simulink model "tiremodel_TUM"  (R2018b)
settings: configuration reference "Physics" (kept outside this file)
model workspace (MAT data in the model file):
  x0_initialstates = Simulink.Parameter
  x0_initialstates.Value = [0 0 0 0 0 0]
  x0_initialstates.DataType = 'auto'
  x0_initialstates.Dimensions = [1 6]
settings Model: DataDictionary=vehicleparameters_vehdynsim.sldd  ParameterArgumentNames=x0_initialstates  OrderedModelArguments=off  Creator=wischnewski  LastModifiedBy=ga25xiw

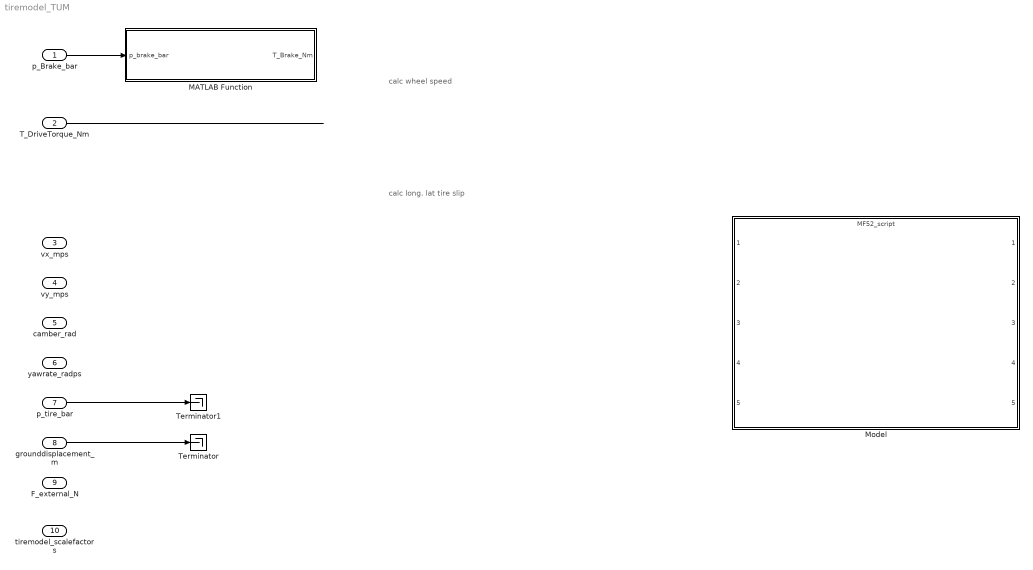
== system tiremodel_TUM ==
  note: calc wheel speed
  note: calc long. lat tire slip
  p_Brake_bar : Inport
  T_DriveTorque_Nm : Inport  Port=2
  vx_mps : Inport  Port=3
  vy_mps : Inport  Port=4
  camber_rad : Inport  Port=5
  yawrate_radps : Inport  Port=6
  p_tire_bar : Inport  Port=7
  grounddisplacement_m : Inport  Port=8
  F_external_N : Inport  Port=9
  tiremodel_scalefactors : Inport  Port=10
  MATLAB Function : MATLAB Function  TreatAsAtomicUnit=on
  Model : ModelReference  ModelNameDialog=MF52_script.slx  SimulationMode=Normal  ModelReferenceVersion=1.5
  Terminator : Terminator
  Terminator1 : Terminator
  wires:
  grounddisplacement_m/1 -> Terminator/1
  p_tire_bar/1 -> Terminator1/1
  p_Brake_bar/1 -> MATLAB Function/1(p_brake_bar)
  T_DriveTorque_Nm/1 -> ?

== matlab function tiremodel_TUM/MATLAB Function ==
  data: p_brake_bar input; T_Brake_Nm output
function T_Brake_Nm = calc_braketorque_wrapper(p_brake_bar)
    
    p_brake_bar
    T_Brake_Nm = 1;
